simulink model "bldc_9"  (R2020a)
settings: Solver=VariableStepAuto  StartTime=0.0  StopTime=3  RelTol=1e-3
PostLoadFcn:
  | kt=0.0275
  | ke=0.0275
model workspace (MAT data in the model file):
  Param = Simulink.Parameter
  Param.DataType = 'auto'
  Param.Dimensions = [0 0]
libraries: simulink x1
settings Model: Creator=I3  LastModifiedBy=I3

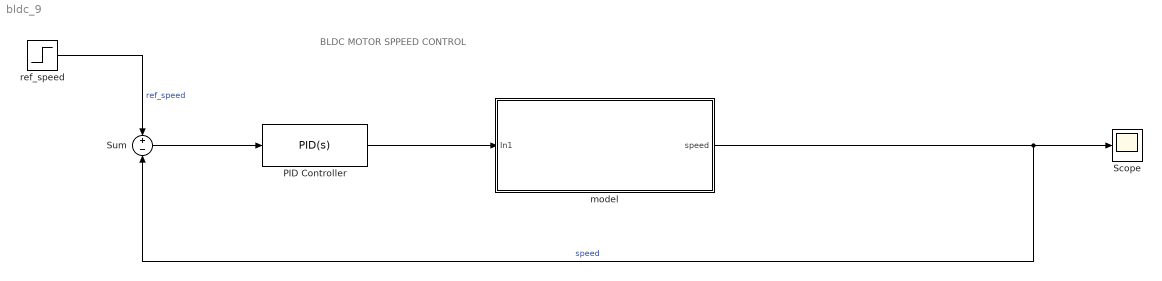
== system bldc_9 ==
  note: BLDC MOTOR SPPEED CONTROL
  PID Controller : simulink/Continuous/PID Controller  Controller=PID  Form=Parallel  TimeDomain=Continuous-time  UseExternalTs=off  SampleTime=-1  IntegratorMethod=Forward Euler  FilterMethod=Forward Euler  ControllerParametersSource=internal  P=0.0192023653437092  I=1.66572762914282  D=4.82616056484106e-05  UseFilter=on  N=83026.6206508631  TunerSelectOption=Transfer Function Based (PID Tuner App)  InitialConditionSource=internal  InitialConditionForIntegrator=0  InitialConditionForFilter=0  DifferentiatorICPrevScaledInput=0  ExternalReset=none  TrackingMode=off  Kt=1  LimitOutput=off  UpperSaturationLimit=inf  LowerSaturationLimit=-inf  LinearizeAsGain=on  AntiWindupMode=none  Kb=1  POutMin=[]  POutMax=[]  IOutMin=[]  IOutMax=[]  DOutMin=[]  DOutMax=[]  NOutMin=[]  NOutMax=[]  SumOutMin=[]  SumOutMax=[]  SaturationOutMin=[]  SaturationOutMax=[]  PParamMin=[]  PParamMax=[]  IParamMin=[]  IParamMax=[]  DParamMin=[]  DParamMax=[]  NParamMin=[]  NParamMax=[]  KbParamMin=[]  KbParamMax=[]  KtParamMin=[]  KtParamMax=[]  KbOutMin=[]  KbOutMax=[]  KtOutMin=[]  KtOutMax=[]  IntegratorOutMin=[]  IntegratorOutMax=[]  FilterOutMin=[]  FilterOutMax=[]  SumI1OutMin=[]  SumI1OutMax=[]  SumI2OutMin=[]  SumI2OutMax=[]  SumI3OutMin=[]  SumI3OutMax=[]  SumI4OutMin=[]  SumI4OutMax=[]  SumDOutMin=[]  SumDOutMax=[]  DifferentiatorOutMin=[]  DifferentiatorOutMax=[]  FilterDiffOutCoefMin=[]  FilterDiffOutCoefMax=[]  ReciprocalOutMin=[]  ReciprocalOutMax=[]  SumDenOutMin=[]  SumDenOutMax=[]  SumNumOutMin=[]  SumNumOutMax=[]  DivideOutMin=[]  DivideOutMax=[]  UdiffTsProdOutMin=[]  UdiffTsProdOutMax=[]  NTsProdOutMin=[]  NTsProdOutMax=[]  UintegralTsProdOutMin=[]  UintegralTsProdOutMax=[]  UngainTsProdOutMin=[]  UngainTsProdOutMax=[]  IntegratorContinuousStateAttributes=''  IntegratorStateMustResolveToSignalObject=off  IntegratorRTWStateStorageClass=Auto  FilterContinuousStateAttributes=''  FilterStateMustResolveToSignalObject=off  FilterRTWStateStorageClass=Auto  ParallelPVariant=InternalParameters  IdealPVariant=Disabled  IVariant=InternalParameters  DVariant=InternalParameters  IntegratorVariant=Continuous  SatVariant=Disabled  AWVariant=Passthrough  PCopyVariant=Disabled  TRVariant=Disabled  FdbkBlocksVariant=Forward  IdealPFdbkVariant=Disabled  SatFdbkVariant=Disabled  DerivativeFilterVariant=ContFilter  NVariant=InternalParameters  NCopyVariant=Disabled  FilterICVariant=InternalICsFilter  IntegratorICVariant=InternalICs  ExternalResetVariant=Disabled  TRSumVariant=Passthrough  SumFdbkVariant=Disabled  SumVariant=Sum_PID  TsampFilterVariant=InternalTs  TsampNgainVariant=Passthrough  TsampIntegralVariant=Passthrough
  Scope : Scope
  Sum : Sum  Inputs=+-
  "model " : Subsystem
  ref_speed : Step  After=1500  SampleTime=0
  wires:
  ref_speed/1 -> Sum/1  "ref_speed"
  Sum/1 -> PID Controller/1
  "model "/1(speed) -> Sum/2, Scope/1  "speed"
  PID Controller/1 -> "model "/1(In1)

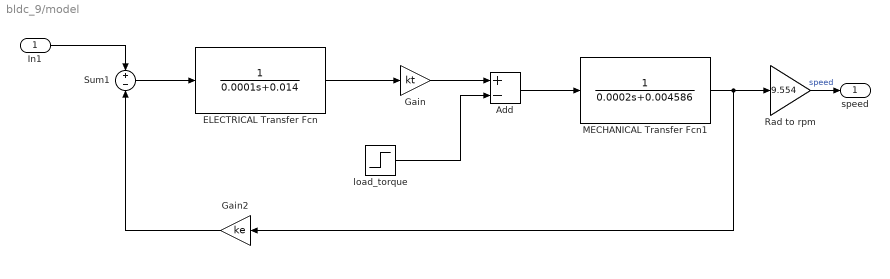
== system bldc_9/model  ==
  In1 : Inport
  Add : Sum  Inputs=+-
  ELECTRICAL Transfer Fcn : TransferFcn  Denominator=[0.0001 0.014]
  Gain : Gain  Gain=kt
  Gain2 : Gain  Gain=ke
  MECHANICAL Transfer Fcn1 : TransferFcn  Denominator=[0.0002 0.004586]
  Rad to rpm : Gain  Gain=9.554
  Sum1 : Sum  Inputs=+-
  load_torque : Step  After=10  SampleTime=0
  speed : Outport
  wires:
  ELECTRICAL Transfer Fcn/1 -> Gain/1
  MECHANICAL Transfer Fcn1/1 -> Gain2/1, Rad to rpm/1
  load_torque/1 -> Add/2
  Sum1/1 -> ELECTRICAL Transfer Fcn/1
  In1/1 -> Sum1/1
  Rad to rpm/1 -> speed/1  "speed"
  Gain/1 -> Add/1
  Gain2/1 -> Sum1/2
  Add/1 -> MECHANICAL Transfer Fcn1/1
